simulink model "QuadcopterSimModel_LindiCopter"  (R2018b)
settings: Solver=ode23  StartTime=0.0  StopTime=1000  FixedStep=sample_time  RelTol=1e-4  EnableMultiTasking=on
undefined symbols (not defined in the file): alt_ground, atmosphere, envir, g, joystick, pos_ref, waypoints, wind
libraries: unit_conversions_lib x3, aerolibfltsims x2, axes_transformation_lib x2, atmosphere_lib x1, lindiCopter_lib x1, sensors_lib x1, quadcopter_lib x1, simulink x1, flightgear_visualization_lib x1, joystick_lib x1
settings Model: EnablePacing=on  Creator=Yannic  LastModifiedBy=yannic
settings SolverCC: ZeroCrossControl=DisableAll
settings DataIOCC: LimitDataPoints=on  ReturnWorkspaceOutputs=on
settings OptimizationCC: EfficientMapNaN2IntZero=off  LifeSpan=inf
settings DebuggingCC: ReadBeforeWriteMsg=DisableAll  WriteAfterWriteMsg=DisableAll  WriteAfterReadMsg=DisableAll  MultiTaskDSMMsg=none  AllowSymbolicDim=off  LibraryContextMissingDiagnostic=none  SFUnexpectedBacktrackingDiag=warning  SFNoUnconditionalDefaultTransitionDiag=warning  SFExecutionAtInitializationDiag=none
settings HardwareCC: TargetBitPerLong=64  TargetBitPerPointer=64  TargetBitPerSizeT=64  TargetBitPerPtrDiffT=64  TargetLongLongMode=on  TargetIntDivRoundTo=Zero  TargetEndianess=LittleEndian  TargetWordSize=64  TargetHWDeviceType=MATLAB Host  ProdEqTarget=off
settings ModelReferenceCC: UpdateModelReferenceTargets=IfOutOfDate  PropagateSignalLabelsOutOfModel=off
settings SFSimCC: SFSimEcho=off  SimUseLocalCustomCode=off
settings CodeAppCC: MaxIdLength=128
settings GRTTargetCC: TargetLangStandard=C89/C90 (ANSI)  CombineOutputUpdateFcns=off  GRTInterface=on
settings ConfigComp: CovMetricSettings=dw  CovHtmlReporting=on  CovSaveCumulativeToWorkspaceVar=on  CovSaveSingleToWorkspaceVar=on  CovExternalEMLEnable=off

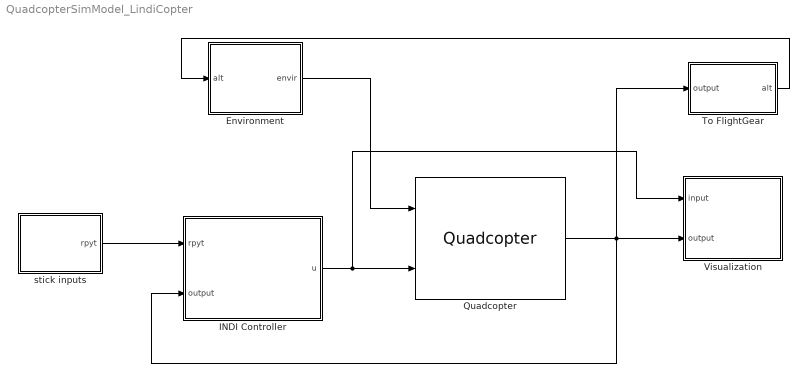
== system QuadcopterSimModel_LindiCopter ==
  Environment : Subsystem
  INDI Controller : Subsystem
  Quadcopter : quadcopter_lib/Quadcopter  copter_=copter  IC_=IC  grnd_=grnd
      settings: SourceProductName=LADAC
  To FlightGear : Subsystem
  Visualization : Subsystem
  stick inputs : Subsystem
  wires:
  Environment/1(envir) -> Quadcopter/1
  Quadcopter/1 -> To FlightGear/1(output), Visualization/2(output), INDI Controller/2(output)
  To FlightGear/1(alt) -> Environment/1(alt)
  INDI Controller/1(u) -> Quadcopter/2, Visualization/1(input)
  stick inputs/1(rpyt) -> INDI Controller/1(rpyt)

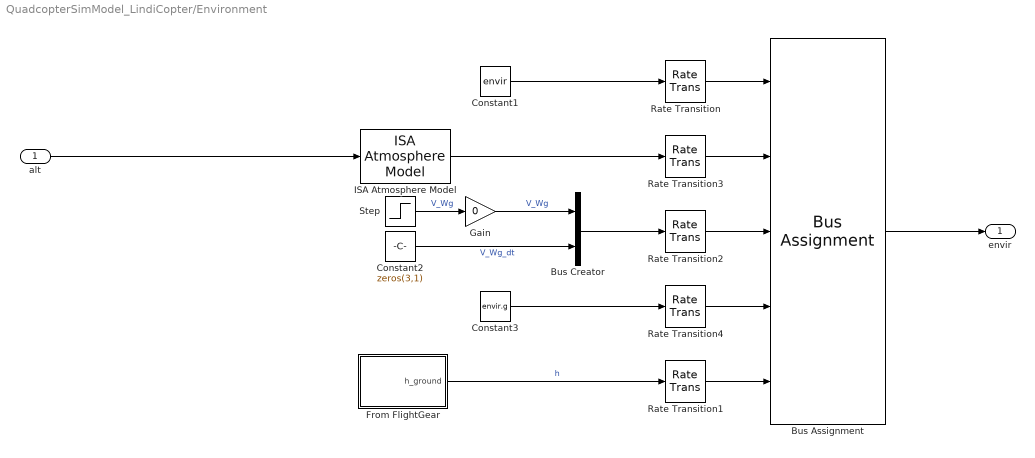
== system QuadcopterSimModel_LindiCopter/Environment ==
  alt : Inport
  Bus Assignment : BusAssignment  AssignedSignals=atmosphere,wind,g,alt_ground
  Bus Creator : BusCreator  Inputs=2
  Constant1 : Constant  Value=envir  OutDataTypeStr=Bus: envirBus
  Constant2 : Constant  Value=zeros(3,1)
  Constant3 : Constant  Value=envir.g
  From FlightGear : Subsystem
  Gain : Gain  Gain=0
  ISA Atmosphere Model : atmosphere_lib/ISA Atmosphere Model
      settings: SourceProductName=LADAC
  Rate Transition{,1..4} (5 alike) : RateTransition
  Step : Step  Time=5  After=[0;10;0]  SampleTime=0
  envir : Outport
  wires:
  From FlightGear/1(h_ground) -> Rate Transition1/1  "h"
  Rate Transition2/1 -> Bus Assignment/3
  Rate Transition3/1 -> Bus Assignment/2
  Bus Assignment/1 -> envir/1
  Rate Transition/1 -> Bus Assignment/1
  ISA Atmosphere Model/1 -> Rate Transition3/1
  Step/1 -> Gain/1  "V_Wg"
  Rate Transition1/1 -> Bus Assignment/5
  Constant1/1 -> Rate Transition/1
  alt/1 -> ISA Atmosphere Model/1
  Bus Creator/1 -> Rate Transition2/1
  Constant2/1 -> Bus Creator/2  "V_Wg_dt"
  Rate Transition4/1 -> Bus Assignment/4
  Constant3/1 -> Rate Transition4/1
  Gain/1 -> Bus Creator/1  "V_Wg"

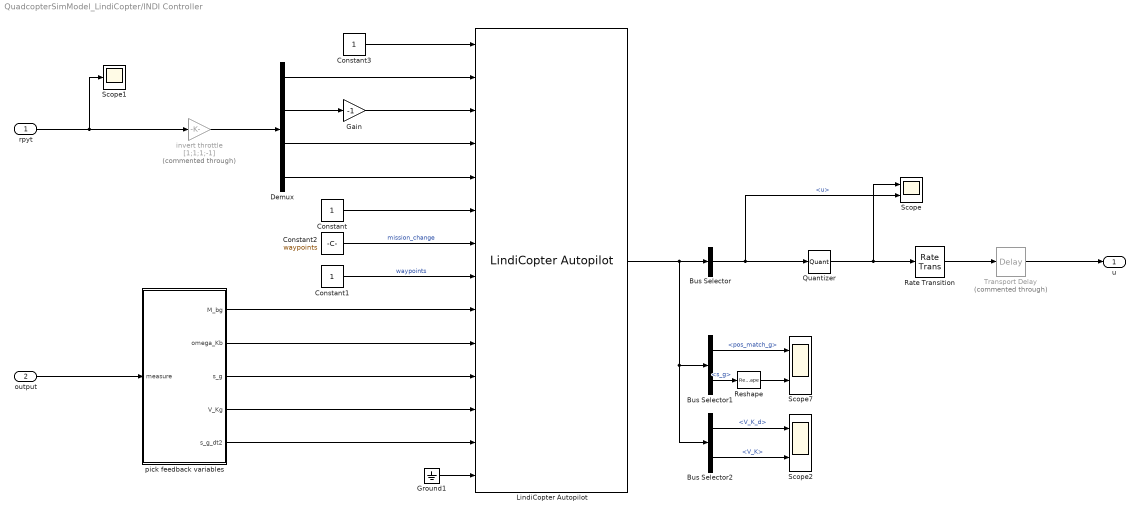
== system QuadcopterSimModel_LindiCopter/INDI Controller ==
  rpyt : Inport  OutDataTypeStr=double
  output : Inport  Port=2
  Bus Selector : BusSelector  OutputSignals=inner_loop_indi.u
  Bus Selector1 : BusSelector  OutputSignals=guidance.matching.pos_match_g,pos_cntrl.measure.s_g
  Bus Selector2 : BusSelector  OutputSignals=guidance.velocity.V_K_d,guidance.velocity.V_K
  Constant : Constant
  Constant1 : Constant
  Constant2 : Constant  Value=waypoints
  Constant3 : Constant
  Demux : Demux
  Gain : Gain  Gain=-1
  Ground1 : Ground
  LindiCopter Autopilot : lindiCopter_lib/LindiCopter Autopilot  ap=lindi
  Quantizer : Quantizer  QuantizationInterval=0.001
  Rate Transition : RateTransition
  Reshape : Reshape
  Scope : Scope  NumInputPorts=2
  Scope1 : Scope
  Scope2 : Scope  NumInputPorts=2
  Scope7 : Scope  NumInputPorts=2
  Transport Delay : TransportDelay  Commented=through  DelayTime=0.0025*0
  invert throttle : Gain  Commented=through  Gain=[1;1;1;-1]
  pick feedback variables : Subsystem
  u : Outport  OutDataTypeStr=double  PortDimensions=4
  wires:
  output/1 -> pick feedback variables/1(measure)
  rpyt/1 -> invert throttle/1, Scope1/1
  Bus Selector/1 -> Quantizer/1, Scope/2  "<u>"
  Transport Delay/1 -> u/1
  invert throttle/1 -> Demux/1
  LindiCopter Autopilot/1 -> Bus Selector2/1, Bus Selector1/1, Bus Selector/1
  Demux/4 -> LindiCopter Autopilot/5
  Demux/3 -> LindiCopter Autopilot/4
  Constant/1 -> LindiCopter Autopilot/6
  Ground1/1 -> LindiCopter Autopilot/14
  Demux/2 -> Gain/1
  Demux/1 -> LindiCopter Autopilot/2
  Gain/1 -> LindiCopter Autopilot/3
  pick feedback variables/1(M_bg) -> LindiCopter Autopilot/9
  pick feedback variables/2(omega_Kb) -> LindiCopter Autopilot/10
  pick feedback variables/3(s_g) -> LindiCopter Autopilot/11
  pick feedback variables/4(V_Kg) -> LindiCopter Autopilot/12
  Constant1/1 -> LindiCopter Autopilot/8  "waypoints"
  Constant2/1 -> LindiCopter Autopilot/7  "mission_change"
  Bus Selector1/2 -> Reshape/1  "<s_g>"
  Bus Selector1/1 -> Scope7/1  "<pos_match_g>"
  Bus Selector2/2 -> Scope2/2  "<V_K>"
  Bus Selector2/1 -> Scope2/1  "<V_K_d>"
  Constant3/1 -> LindiCopter Autopilot/1
  Quantizer/1 -> Rate Transition/1, Scope/1
  pick feedback variables/5(s_g_dt2) -> LindiCopter Autopilot/13
  Rate Transition/1 -> Transport Delay/1
  Reshape/1 -> Scope7/2

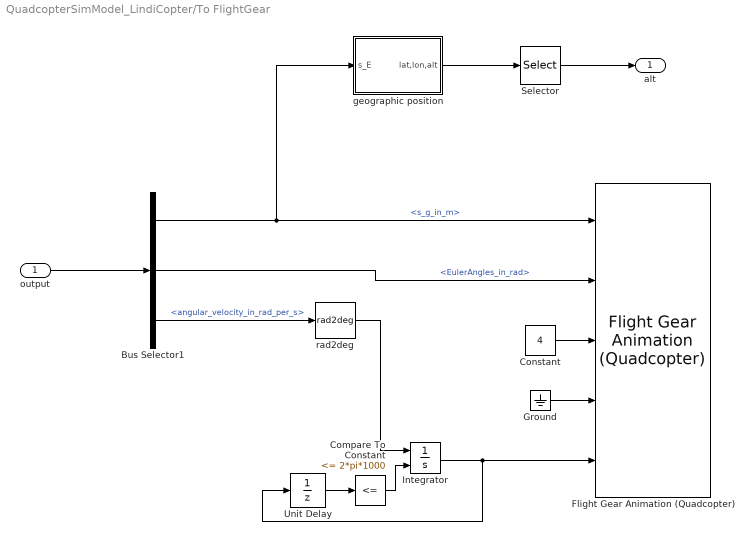
== system QuadcopterSimModel_LindiCopter/To FlightGear ==
  output : Inport
  Bus Selector1 : BusSelector  OutputSignals=rigidBodyBus.s_g_in_m,rigidBodyBus.EulerAngles_in_rad,motorBus.angular_velocity_in_rad_per_s
  Compare To Constant : simulink/Logic and Bit Operations/Compare To Constant  relop=<=  const=2*pi*1000  OutDataTypeStr=boolean
  Constant : Constant  Value=4
  Flight Gear Animation (Quadcopter) : flightgear_visualization_lib/Flight Gear Animation (Quadcopter)  inital_lat=pos_ref.lat  inital_long=pos_ref.lon  inital_height=pos_ref.alt  remoteURL=fg.remoteURL  remotePort=fg.remotePort
      settings: SourceProductName=LADAC
  Ground : Ground
  Integrator : Integrator  ExternalReset=rising
  Selector : Selector  InputPortWidth=3  IndexOptions=Index vector (dialog)  Indices=3  OutputSizes=1
  Unit Delay : UnitDelay  SampleTime=-1
  geographic position : Subsystem
  rad2deg : unit_conversions_lib/rad2deg
      settings: SourceProductName=LADAC
  alt : Outport
  wires:
  Bus Selector1/1 -> geographic position/1(s_E), Flight Gear Animation (Quadcopter)/1  "<s_g_in_m>"
  output/1 -> Bus Selector1/1
  geographic position/1(lat,lon,alt) -> Selector/1
  Bus Selector1/2 -> Flight Gear Animation (Quadcopter)/2  "<EulerAngles_in_rad>"
  Bus Selector1/3 -> rad2deg/1  "<angular_velocity_in_rad_per_s>"
  Selector/1 -> alt/1
  Constant/1 -> Flight Gear Animation (Quadcopter)/3
  Ground/1 -> Flight Gear Animation (Quadcopter)/4
  Integrator/1 -> Unit Delay/1, Flight Gear Animation (Quadcopter)/5
  Unit Delay/1 -> Compare To Constant/1
  Compare To Constant/1 -> Integrator/2
  rad2deg/1 -> Integrator/1

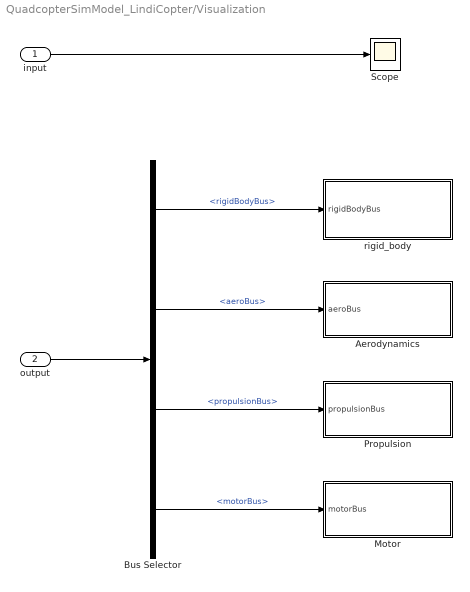
== system QuadcopterSimModel_LindiCopter/Visualization ==
  input : Inport
  output : Inport  Port=2
  Aerodynamics : Subsystem
  Bus Selector : BusSelector  OutputSignals=rigidBodyBus,aeroBus,propulsionBus,motorBus
  Motor : Subsystem
  Propulsion : Subsystem
  Scope : Scope
  rigid_body : Subsystem
  wires:
  output/1 -> Bus Selector/1
  Bus Selector/1 -> rigid_body/1(rigidBodyBus)  "<rigidBodyBus>"
  Bus Selector/2 -> Aerodynamics/1(aeroBus)  "<aeroBus>"
  Bus Selector/3 -> Propulsion/1(propulsionBus)  "<propulsionBus>"
  Bus Selector/4 -> Motor/1(motorBus)  "<motorBus>"
  input/1 -> Scope/1

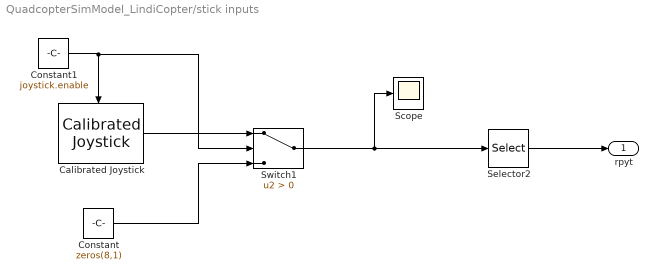
== system QuadcopterSimModel_LindiCopter/stick inputs ==
  Calibrated Joystick : joystick_lib/Calibrated Joystick  jystck=joystick
      settings: SourceProductName=LADAC
  Constant : Constant  Value=zeros(8,1)
  Constant1 : Constant  Value=joystick.enable
  Scope : Scope
  Selector2 : Selector  InputPortWidth=8  IndexOptions=Index vector (dialog)  Indices=[1,2,3,4]  OutputSizes=1
  Switch1 : Switch  Criteria=u2 > Threshold
  rpyt : Outport
  wires:
  Constant/1 -> Switch1/3
  Switch1/1 -> Selector2/1, Scope/1
  Constant1/1 -> Calibrated Joystick/Enable, Switch1/2
  Calibrated Joystick/1 -> Switch1/1
  Selector2/1 -> rpyt/1

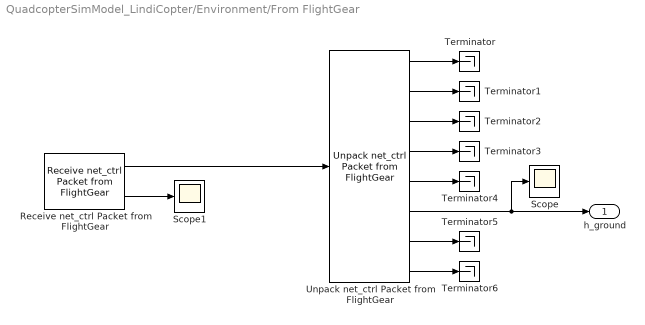
== system QuadcopterSimModel_LindiCopter/Environment/From FlightGear ==
  Receive net_ctrl Packet from FlightGear : aerolibfltsims/Receive net_ctrl Packet from FlightGear  FlightGearVersion=v3.4  ReceiveAddress=127.0.0.1  ReceivePort=5503  ReceiveWidth=744  varLen=off  SampleTime=1/5  packetFlag=on
      settings: AttributesFormatString=Version Selected:\n%<FlightGearVersion>  SourceProductName=Aerospace Blockset  SourceProductBaseCode=AE
  Scope : Scope
  Scope1 : Scope
  Terminator{,1..6} (7 alike) : Terminator
  Unpack net_ctrl Packet from FlightGear : aerolibfltsims/Unpack net_ctrl Packet from FlightGear  FlightGearVersion=v3.4  ShowControlSurfacePositionOutputs=off  ShowEngineFuelOutputs=off  ShowLandingGearOutputs=off  ShowAvionicOutputs=off  ShowEnvironmentOutputs=on  SampleTime=1/5  packetVersion=27
      settings: AttributesFormatString=Version Selected: %<FlightGearVersion>  SourceProductName=Aerospace Blockset  SourceProductBaseCode=AE
  h_ground : Outport
  wires:
  Unpack net_ctrl Packet from FlightGear/4 -> Terminator3/1
  Unpack net_ctrl Packet from FlightGear/5 -> Terminator4/1
  Receive net_ctrl Packet from FlightGear/1 -> Unpack net_ctrl Packet from FlightGear/1
  Unpack net_ctrl Packet from FlightGear/2 -> Terminator1/1
  Unpack net_ctrl Packet from FlightGear/7 -> Terminator5/1
  Unpack net_ctrl Packet from FlightGear/1 -> Terminator/1
  Unpack net_ctrl Packet from FlightGear/3 -> Terminator2/1
  Unpack net_ctrl Packet from FlightGear/8 -> Terminator6/1
  Unpack net_ctrl Packet from FlightGear/6 -> Scope/1, h_ground/1
  Receive net_ctrl Packet from FlightGear/2 -> Scope1/1

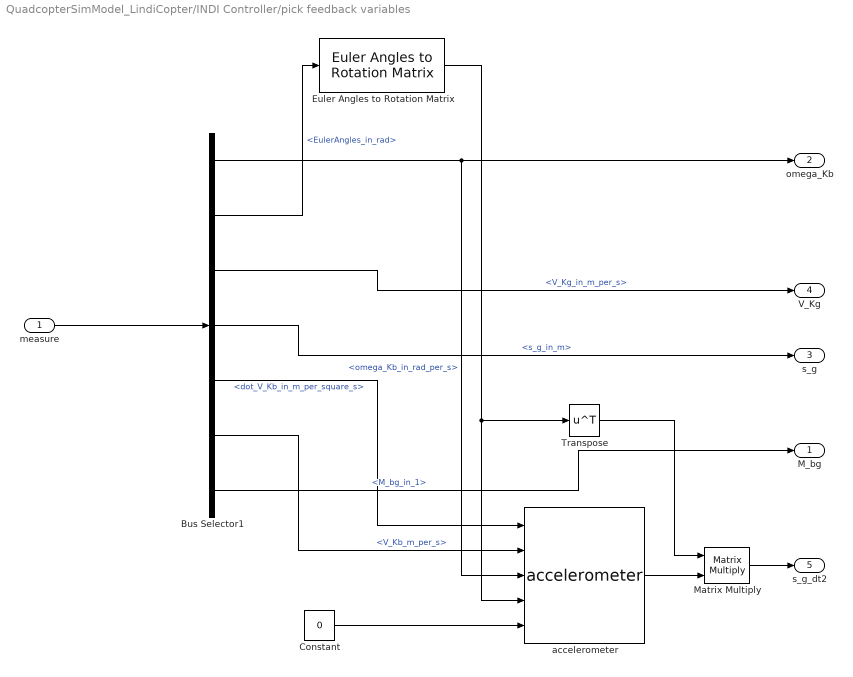
== system QuadcopterSimModel_LindiCopter/INDI Controller/pick feedback variables ==
  measure : Inport
  Bus Selector1 : BusSelector  OutputSignals=rigidBodyBus.omega_Kb_in_rad_per_s,rigidBodyBus.EulerAngles_in_rad,rigidBodyBus.V_Kg_in_m_per_s,rigidBodyBus.s_g_in_m,rigidBodyBus.dot_V_Kb_in_m_per_square_s,rigidBodyBus.V_Kb_m_per_s,rigidBodyBus.M_bg_in_1
  Constant : Constant  Value=0  OutDataTypeStr=Inherit: Inherit via back propagation
  Euler Angles to Rotation Matrix : axes_transformation_lib/Euler Angles to Rotation Matrix  SystemSampleTime=-1
      settings: SourceProductName=LADAC
  Matrix Multiply : Product  Multiplication=Matrix(*)
  Transpose : Math  Operator=transpose  SaturateOnIntegerOverflow=on
  accelerometer : sensors_lib/accelerometer  SystemSampleTime=-1
      settings: SourceProductName=LADAC
  M_bg : Outport
  omega_Kb : Outport  Port=2
  s_g : Outport  Port=3
  V_Kg : Outport  Port=4
  s_g_dt2 : Outport  Port=5
  wires:
  measure/1 -> Bus Selector1/1
  Bus Selector1/3 -> V_Kg/1  "<V_Kg_in_m_per_s>"
  Bus Selector1/2 -> Euler Angles to Rotation Matrix/1  "<EulerAngles_in_rad>"
  Bus Selector1/1 -> omega_Kb/1, accelerometer/3  "<omega_Kb_in_rad_per_s>"
  Bus Selector1/4 -> s_g/1  "<s_g_in_m>"
  Bus Selector1/5 -> accelerometer/1  "<dot_V_Kb_in_m_per_square_s>"
  Euler Angles to Rotation Matrix/1 -> accelerometer/4, Transpose/1
  Bus Selector1/6 -> accelerometer/2  "<V_Kb_m_per_s>"
  Constant/1 -> accelerometer/5
  accelerometer/1 -> Matrix Multiply/2
  Matrix Multiply/1 -> s_g_dt2/1
  Transpose/1 -> Matrix Multiply/1
  Bus Selector1/7 -> M_bg/1  "<M_bg_in_1>"

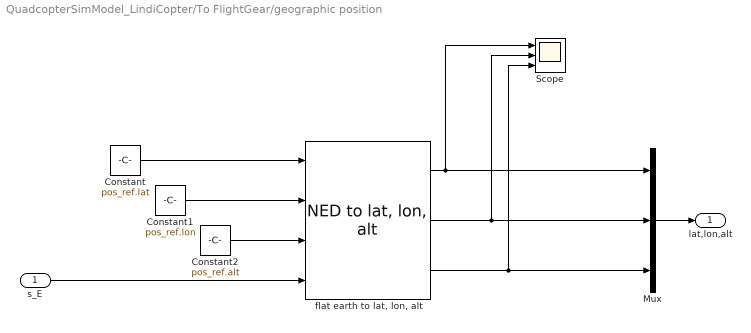
== system QuadcopterSimModel_LindiCopter/To FlightGear/geographic position ==
  s_E : Inport
  Constant : Constant  Value=pos_ref.lat
  Constant1 : Constant  Value=pos_ref.lon
  Constant2 : Constant  Value=pos_ref.alt
  Mux : Mux  Inputs=3
  Scope : Scope  NumInputPorts=3
  "flat earth to lat, lon, alt" : axes_transformation_lib/NED to lat, lon, alt  SystemSampleTime=-1
      settings: SourceProductName=LADAC
  lat,lon,alt : Outport
  wires:
  Constant2/1 -> "flat earth to lat, lon, alt"/3
  Constant1/1 -> "flat earth to lat, lon, alt"/2
  "flat earth to lat, lon, alt"/3 -> Scope/3, Mux/3
  Constant/1 -> "flat earth to lat, lon, alt"/1
  Mux/1 -> lat,lon,alt/1
  s_E/1 -> "flat earth to lat, lon, alt"/4
  "flat earth to lat, lon, alt"/2 -> Mux/2, Scope/2
  "flat earth to lat, lon, alt"/1 -> Mux/1, Scope/1

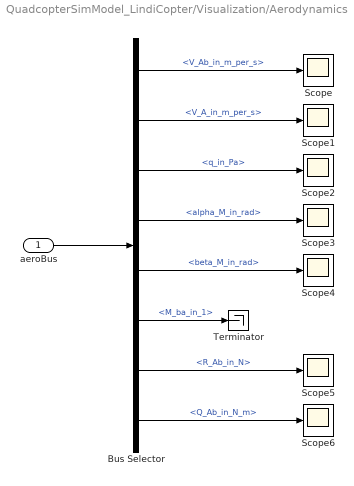
== system QuadcopterSimModel_LindiCopter/Visualization/Aerodynamics ==
  aeroBus : Inport
  Bus Selector : BusSelector  OutputSignals=V_Ab_in_m_per_s,V_A_in_m_per_s,q_in_Pa,angles.alpha_M_in_rad,angles.beta_M_in_rad,M_ba_in_1,R_Ab_in_N,Q_Ab_in_N_m
  Scope{,1..6} (7 alike) : Scope
  Terminator : Terminator
  wires:
  aeroBus/1 -> Bus Selector/1
  Bus Selector/1 -> Scope/1  "<V_Ab_in_m_per_s>"
  Bus Selector/2 -> Scope1/1  "<V_A_in_m_per_s>"
  Bus Selector/3 -> Scope2/1  "<q_in_Pa>"
  Bus Selector/4 -> Scope3/1  "<alpha_M_in_rad>"
  Bus Selector/5 -> Scope4/1  "<beta_M_in_rad>"
  Bus Selector/6 -> Terminator/1  "<M_ba_in_1>"
  Bus Selector/7 -> Scope5/1  "<R_Ab_in_N>"
  Bus Selector/8 -> Scope6/1  "<Q_Ab_in_N_m>"

== system QuadcopterSimModel_LindiCopter/Visualization/Motor ==
  motorBus : Inport
  Bus Selector : BusSelector  OutputSignals=angular_acceleration_in_rad_per_square_s,angular_velocity_in_rad_per_s
  Scope : Scope
  Scope1 : Scope
  wires:
  Bus Selector/1 -> Scope/1  "<angular_acceleration_in_rad_per_square_s>"
  motorBus/1 -> Bus Selector/1
  Bus Selector/2 -> Scope1/1  "<angular_velocity_in_rad_per_s>"

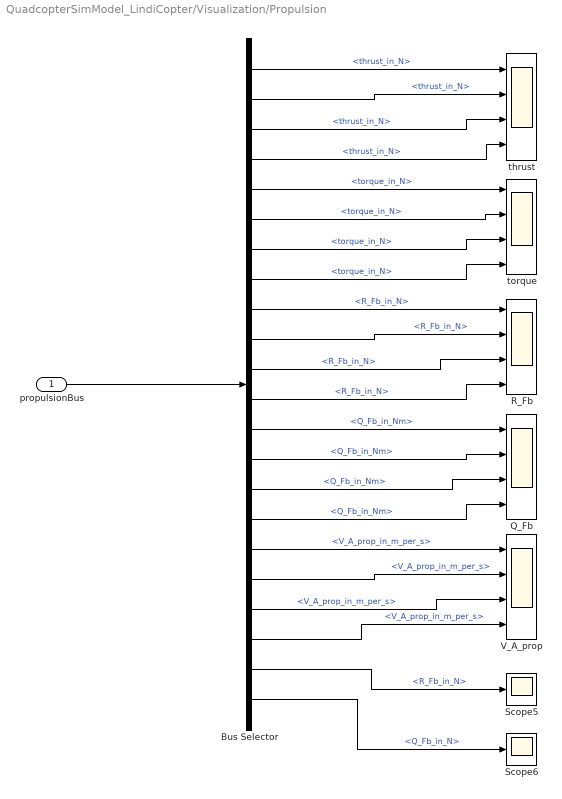
== system QuadcopterSimModel_LindiCopter/Visualization/Propulsion ==
  propulsionBus : Inport
  Bus Selector : BusSelector  OutputSignals=propeller_1.thrust_in_N,propeller_2.thrust_in_N,propeller_3.thrust_in_N,propeller_4.thrust_in_N,propeller_1.torque_in_N,propeller_2.torque_in_N,propeller_3.torque_in_N,propeller_4.torque_in_N,propeller_1.R_Fb_in_N,propeller_2.R_Fb_in_N,propeller_3.R_Fb_in_N,propeller_4.R_Fb_in_N,propeller_1.Q_Fb_in_Nm,propeller_2.Q_Fb_in_Nm,propeller_3.Q_Fb_in_Nm,propeller_4.Q_Fb_in_Nm,propeller_1.V_A_prop_in_m_per_s,propeller_2.V_A_prop_in_m_per_s,propeller_3.V_A_prop_in_m_per_s,propeller_4.V_A_prop_in_m_per_s,R_Fb_in_N,Q_Fb_in_N
  Q_Fb : Scope  NumInputPorts=4
  R_Fb : Scope  NumInputPorts=4
  Scope5 : Scope
  Scope6 : Scope
  V_A_prop : Scope  NumInputPorts=4
  thrust : Scope  NumInputPorts=4
  torque : Scope  NumInputPorts=4
  wires:
  propulsionBus/1 -> Bus Selector/1
  Bus Selector/1 -> thrust/1  "<thrust_in_N>"
  Bus Selector/2 -> thrust/2  "<thrust_in_N>"
  Bus Selector/3 -> thrust/3  "<thrust_in_N>"
  Bus Selector/4 -> thrust/4  "<thrust_in_N>"
  Bus Selector/5 -> torque/1  "<torque_in_N>"
  Bus Selector/6 -> torque/2  "<torque_in_N>"
  Bus Selector/7 -> torque/3  "<torque_in_N>"
  Bus Selector/8 -> torque/4  "<torque_in_N>"
  Bus Selector/9 -> R_Fb/1  "<R_Fb_in_N>"
  Bus Selector/10 -> R_Fb/2  "<R_Fb_in_N>"
  Bus Selector/11 -> R_Fb/3  "<R_Fb_in_N>"
  Bus Selector/12 -> R_Fb/4  "<R_Fb_in_N>"
  Bus Selector/13 -> Q_Fb/1  "<Q_Fb_in_Nm>"
  Bus Selector/14 -> Q_Fb/2  "<Q_Fb_in_Nm>"
  Bus Selector/15 -> Q_Fb/3  "<Q_Fb_in_Nm>"
  Bus Selector/16 -> Q_Fb/4  "<Q_Fb_in_Nm>"
  Bus Selector/17 -> V_A_prop/1  "<V_A_prop_in_m_per_s>"
  Bus Selector/18 -> V_A_prop/2  "<V_A_prop_in_m_per_s>"
  Bus Selector/19 -> V_A_prop/3  "<V_A_prop_in_m_per_s>"
  Bus Selector/20 -> V_A_prop/4  "<V_A_prop_in_m_per_s>"
  Bus Selector/21 -> Scope5/1  "<R_Fb_in_N>"
  Bus Selector/22 -> Scope6/1  "<Q_Fb_in_N>"

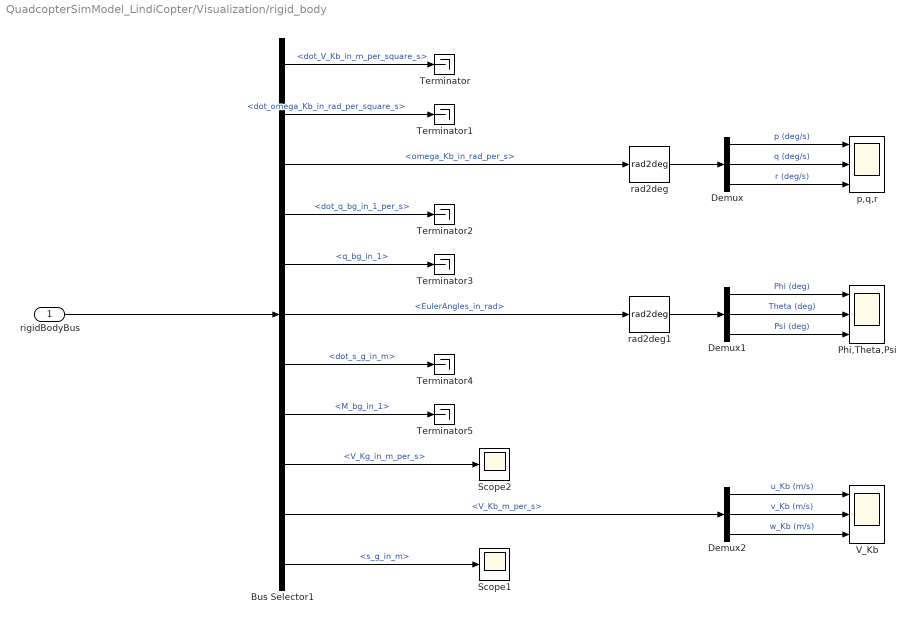
== system QuadcopterSimModel_LindiCopter/Visualization/rigid_body ==
  rigidBodyBus : Inport
  Bus Selector1 : BusSelector  OutputSignals=dot_V_Kb_in_m_per_square_s,dot_omega_Kb_in_rad_per_square_s,omega_Kb_in_rad_per_s,dot_q_bg_in_1_per_s,q_bg_in_1,EulerAngles_in_rad,dot_s_g_in_m,M_bg_in_1,V_Kg_in_m_per_s,V_Kb_m_per_s,s_g_in_m
  Demux : Demux  Outputs=3
  Demux1 : Demux  Outputs=3
  Demux2 : Demux  Outputs=3
  Phi,Theta,Psi : Scope  NumInputPorts=3
  Scope1 : Scope
  Scope2 : Scope
  Terminator{,1..5} (6 alike) : Terminator
  V_Kb : Scope  NumInputPorts=3
  p,q,r : Scope  NumInputPorts=3
  rad2deg : unit_conversions_lib/rad2deg
      settings: SourceProductName=LADAC
  rad2deg1 : unit_conversions_lib/rad2deg
      settings: SourceProductName=LADAC
  wires:
  Demux/1 -> p,q,r/1  "p (deg/s)"
  Demux1/2 -> Phi,Theta,Psi/2  "Theta (deg)"
  rad2deg/1 -> Demux/1
  Demux1/1 -> Phi,Theta,Psi/1  "Phi (deg)"
  Demux1/3 -> Phi,Theta,Psi/3  "Psi (deg)"
  Demux2/3 -> V_Kb/3  "w_Kb (m/s)"
  Bus Selector1/7 -> Terminator4/1  "<dot_s_g_in_m>"
  Bus Selector1/6 -> rad2deg1/1  "<EulerAngles_in_rad>"
  Bus Selector1/3 -> rad2deg/1  "<omega_Kb_in_rad_per_s>"
  Demux/3 -> p,q,r/3  "r (deg/s)"
  Bus Selector1/1 -> Terminator/1  "<dot_V_Kb_in_m_per_square_s>"
  Demux2/2 -> V_Kb/2  "v_Kb (m/s)"
  Demux/2 -> p,q,r/2  "q (deg/s)"
  rad2deg1/1 -> Demux1/1
  Bus Selector1/5 -> Terminator3/1  "<q_bg_in_1>"
  Demux2/1 -> V_Kb/1  "u_Kb (m/s)"
  Bus Selector1/10 -> Demux2/1  "<V_Kb_m_per_s>"
  rigidBodyBus/1 -> Bus Selector1/1
  Bus Selector1/8 -> Terminator5/1  "<M_bg_in_1>"
  Bus Selector1/4 -> Terminator2/1  "<dot_q_bg_in_1_per_s>"
  Bus Selector1/2 -> Terminator1/1  "<dot_omega_Kb_in_rad_per_square_s>"
  Bus Selector1/9 -> Scope2/1  "<V_Kg_in_m_per_s>"
  Bus Selector1/11 -> Scope1/1  "<s_g_in_m>"
